simulink model "8Bit_Register"  (R2019b)
settings: Solver=FixedStepDiscrete  StartTime=0.0  StopTime=10.0  RelTol=1e-3
libraries: hdlsllib x9, simulink_extras x9
settings Model: Creator=cohen  LastModifiedBy=cohen

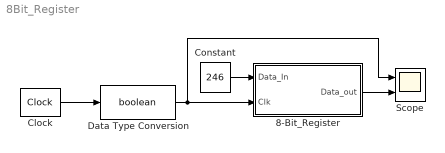
== system 8Bit_Register ==
  8-Bit_Register : Subsystem
  Clock : simulink_extras/Flip Flops/Clock  period=1
  Constant : Constant  Value=246  OutDataTypeStr=uint8  SampleTime=1
  Data Type Conversion : DataTypeConversion  OutDataTypeStr=boolean
  Scope : Scope  NumInputPorts=2
  wires:
  Constant/1 -> 8-Bit_Register/1(Data_In)
  Clock/1 -> Data Type Conversion/1
  Data Type Conversion/1 -> Scope/1, 8-Bit_Register/2(Clk)
  8-Bit_Register/1(Data_out) -> Scope/2

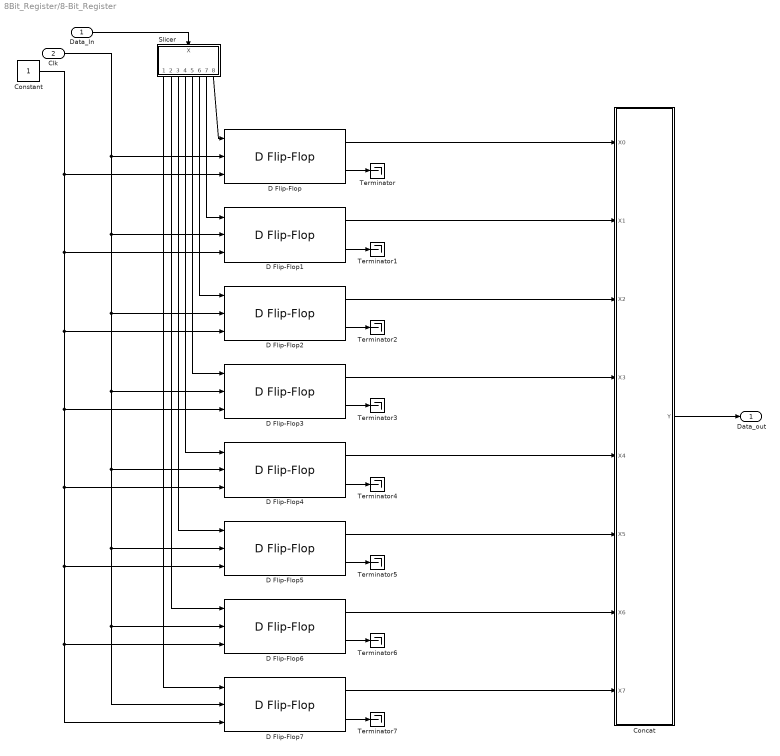
== system 8Bit_Register/8-Bit_Register ==
  Data_In : Inport  OutDataTypeStr=uint8
  Clk : Inport  Port=2
  Concat : Subsystem
  Constant : Constant  OutDataTypeStr=boolean  SampleTime=1
  D Flip-Flop{,1..7} (8 alike) : simulink_extras/Flip Flops/D Flip-Flop
      settings: SourceProductName=Simulink
  Slicer : Subsystem
  Terminator{,1..7} (8 alike) : Terminator
  Data_out : Outport  OutDataTypeStr=uint8
  wires:
  D Flip-Flop6/1 -> Concat/7(X6)
  Slicer/3(Y5) -> D Flip-Flop5/1
  D Flip-Flop5/1 -> Concat/6(X5)
  D Flip-Flop2/1 -> Concat/3(X2)
  Constant/1 -> D Flip-Flop/3, D Flip-Flop2/3, D Flip-Flop3/3, D Flip-Flop4/3, D Flip-Flop5/3, D Flip-Flop6/3, D Flip-Flop7/3, D Flip-Flop1/3
  Clk/1 -> D Flip-Flop/2, D Flip-Flop1/2, D Flip-Flop2/2, D Flip-Flop3/2, D Flip-Flop4/2, D Flip-Flop6/2, D Flip-Flop7/2, D Flip-Flop5/2
  D Flip-Flop4/1 -> Concat/5(X4)
  D Flip-Flop2/2 -> Terminator2/1
  Slicer/5(Y3) -> D Flip-Flop3/1
  Slicer/1(Y7) -> D Flip-Flop7/1
  Concat/1(Y) -> Data_out/1
  D Flip-Flop5/2 -> Terminator5/1
  D Flip-Flop7/1 -> Concat/8(X7)
  Slicer/7(Y1) -> D Flip-Flop1/1
  D Flip-Flop1/1 -> Concat/2(X1)
  D Flip-Flop6/2 -> Terminator6/1
  Slicer/6(Y2) -> D Flip-Flop2/1
  D Flip-Flop3/1 -> Concat/4(X3)
  D Flip-Flop/1 -> Concat/1(X0)
  D Flip-Flop4/2 -> Terminator4/1
  D Flip-Flop3/2 -> Terminator3/1
  D Flip-Flop7/2 -> Terminator7/1
  D Flip-Flop/2 -> Terminator/1
  Slicer/4(Y4) -> D Flip-Flop4/1
  Data_In/1 -> Slicer/1(X)
  Slicer/8(Y0) -> D Flip-Flop/1
  Slicer/2(Y6) -> D Flip-Flop6/1
  D Flip-Flop1/2 -> Terminator1/1

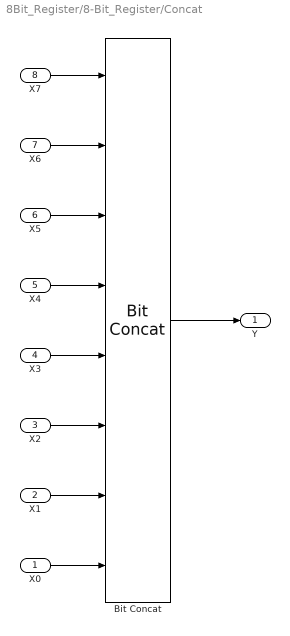
== system 8Bit_Register/8-Bit_Register/Concat ==
  X0 : Inport  OutDataTypeStr=boolean  SampleTime=1
  X1 : Inport  Port=2  OutDataTypeStr=boolean  SampleTime=1
  X2 : Inport  Port=3  OutDataTypeStr=boolean  SampleTime=1
  X3 : Inport  Port=4  OutDataTypeStr=boolean  SampleTime=1
  X4 : Inport  Port=5  OutDataTypeStr=boolean  SampleTime=1
  X5 : Inport  Port=6  OutDataTypeStr=boolean  SampleTime=1
  X6 : Inport  Port=7  OutDataTypeStr=boolean  SampleTime=1
  X7 : Inport  Port=8  OutDataTypeStr=boolean  SampleTime=1
  Bit Concat : hdlsllib/Logic and Bit Operations/Bit Concat  numInputs=8
      settings: SourceProductName=Simulink
  Y : Outport  SampleTime=1
  wires:
  X6/1 -> Bit Concat/2
  X2/1 -> Bit Concat/6
  X7/1 -> Bit Concat/1
  X0/1 -> Bit Concat/8
  Bit Concat/1 -> Y/1
  X3/1 -> Bit Concat/5
  X1/1 -> Bit Concat/7
  X5/1 -> Bit Concat/3
  X4/1 -> Bit Concat/4

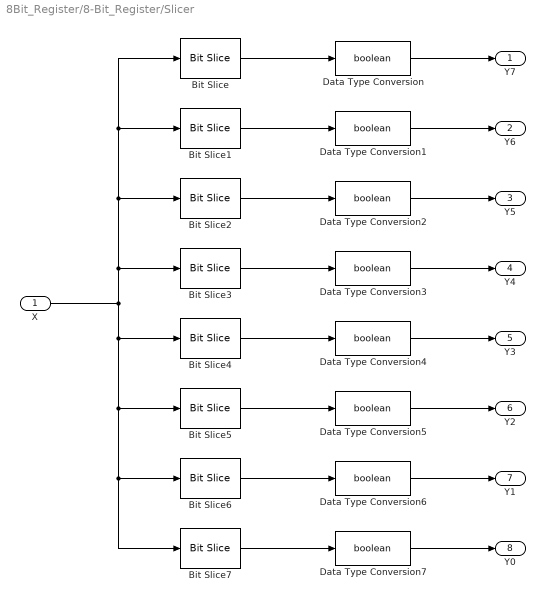
== system 8Bit_Register/8-Bit_Register/Slicer ==
  X : Inport  OutDataTypeStr=uint8  SampleTime=1
  Bit Slice : hdlsllib/Logic and Bit Operations/Bit Slice  lidx=7  ridx=7
      settings: SourceProductName=Simulink  SourceProductBaseCode=SL
  Bit Slice1 : hdlsllib/Logic and Bit Operations/Bit Slice  lidx=6  ridx=6
      settings: SourceProductName=Simulink  SourceProductBaseCode=SL
  Bit Slice2 : hdlsllib/Logic and Bit Operations/Bit Slice  lidx=5  ridx=5
      settings: SourceProductName=Simulink  SourceProductBaseCode=SL
  Bit Slice3 : hdlsllib/Logic and Bit Operations/Bit Slice  lidx=4  ridx=4
      settings: SourceProductName=Simulink  SourceProductBaseCode=SL
  Bit Slice4 : hdlsllib/Logic and Bit Operations/Bit Slice  lidx=3  ridx=3
      settings: SourceProductName=Simulink  SourceProductBaseCode=SL
  Bit Slice5 : hdlsllib/Logic and Bit Operations/Bit Slice  lidx=2  ridx=2
      settings: SourceProductName=Simulink  SourceProductBaseCode=SL
  Bit Slice6 : hdlsllib/Logic and Bit Operations/Bit Slice  lidx=1  ridx=1
      settings: SourceProductName=Simulink  SourceProductBaseCode=SL
  Bit Slice7 : hdlsllib/Logic and Bit Operations/Bit Slice  lidx=0  ridx=0
      settings: SourceProductName=Simulink  SourceProductBaseCode=SL
  Data Type Conversion{,1..7} (8 alike) : DataTypeConversion  OutDataTypeStr=boolean
  Y7 : Outport  OutDataTypeStr=boolean  SampleTime=1
  Y6 : Outport  Port=2  OutDataTypeStr=boolean  SampleTime=1
  Y5 : Outport  Port=3  OutDataTypeStr=boolean  SampleTime=1
  Y4 : Outport  Port=4  OutDataTypeStr=boolean
  Y3 : Outport  Port=5  OutDataTypeStr=boolean  SampleTime=1
  Y2 : Outport  Port=6  OutDataTypeStr=boolean  SampleTime=1
  Y1 : Outport  Port=7  OutDataTypeStr=boolean  SampleTime=1
  Y0 : Outport  Port=8  OutDataTypeStr=boolean  SampleTime=1
  wires:
  Bit Slice6/1 -> Data Type Conversion6/1
  X/1 -> Bit Slice3/1, Bit Slice2/1, Bit Slice1/1, Bit Slice/1, Bit Slice4/1, Bit Slice5/1, Bit Slice6/1, Bit Slice7/1
  Bit Slice/1 -> Data Type Conversion/1
  Bit Slice7/1 -> Data Type Conversion7/1
  Bit Slice4/1 -> Data Type Conversion4/1
  Bit Slice1/1 -> Data Type Conversion1/1
  Bit Slice3/1 -> Data Type Conversion3/1
  Data Type Conversion1/1 -> Y6/1
  Data Type Conversion7/1 -> Y0/1
  Data Type Conversion5/1 -> Y2/1
  Data Type Conversion3/1 -> Y4/1
  Data Type Conversion4/1 -> Y3/1
  Bit Slice2/1 -> Data Type Conversion2/1
  Bit Slice5/1 -> Data Type Conversion5/1
  Data Type Conversion6/1 -> Y1/1
  Data Type Conversion/1 -> Y7/1
  Data Type Conversion2/1 -> Y5/1
